simulink model "start"  (R2022b)
settings: Solver=VariableStepAuto  StartTime=0.0  StopTime=20.00  RelTol=1e-3
settings Model: Creator=Asus Notebook  LastModifiedBy=Asus Notebook

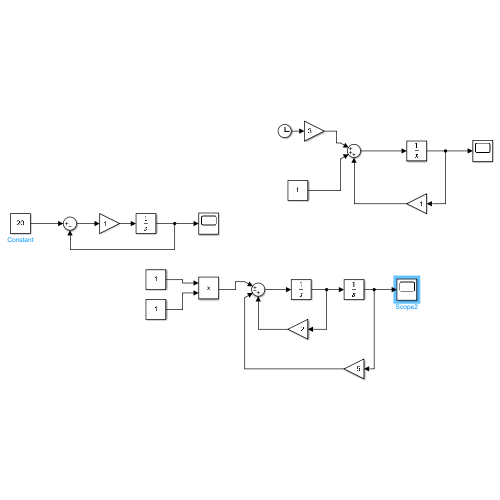
[thumbnail: Simulink's stored preview of the top-level diagram]
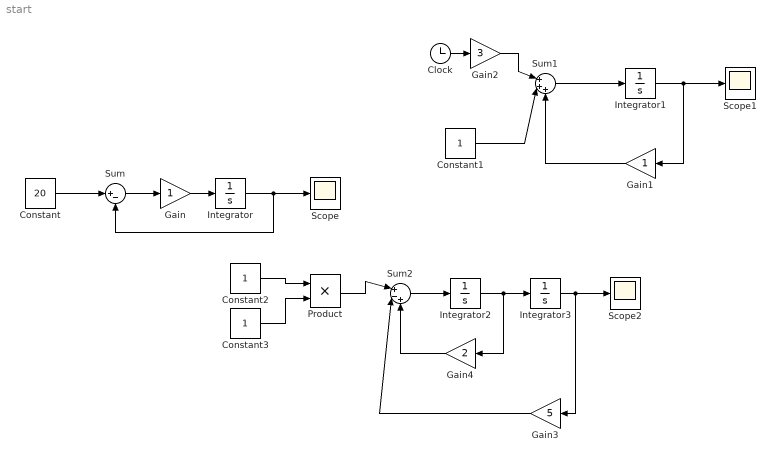
== system start ==
  Clock : Clock
  Constant : Constant  Value=20
  Constant1 : Constant
  Constant2 : Constant
  Constant3 : Constant
  Gain : Gain
  Gain1 : Gain
  Gain2 : Gain  Gain=3
  Gain3 : Gain  Gain=5
  Gain4 : Gain  Gain=2
  Integrator : Integrator  InitialCondition=60
  Integrator1 : Integrator
  Integrator2 : Integrator
  Integrator3 : Integrator
  Product : Product
  Scope : Scope
  Scope1 : Scope
  Scope2 : Scope
  Sum : Sum  Inputs=|+-
  Sum1 : Sum  Inputs=|+++
  Sum2 : Sum  Inputs=|+-+
  wires:
  Constant/1 -> Sum/1
  Sum/1 -> Gain/1
  Gain/1 -> Integrator/1
  Integrator/1 -> Sum/2, Scope/1
  Integrator1/1 -> Gain1/1, Scope1/1
  Gain1/1 -> Sum1/3
  Constant1/1 -> Sum1/2
  Clock/1 -> Gain2/1
  Gain2/1 -> Sum1/1
  Sum1/1 -> Integrator1/1
  Integrator2/1 -> Gain4/1, Integrator3/1
  Integrator3/1 -> Scope2/1, Gain3/1
  Gain3/1 -> Sum2/2
  Sum2/1 -> Integrator2/1
  Gain4/1 -> Sum2/3
  Constant2/1 -> Product/1
  Constant3/1 -> Product/2
  Product/1 -> Sum2/1
